simulink library "INP_UNSP_ManOver"  (R2024b)
settings: Solver=VariableStepAuto  StartTime=0.0  StopTime=10.0  RelTol=1e-3
undefined symbols (not defined in the file): INP_UNSP_p_SwtAccUnspFrLeMan_na, INP_UNSP_p_SwtAccUnspFrRiMan_na, INP_UNSP_p_SwtAccUnspReLeMan_na, INP_UNSP_p_SwtAccUnspReRiMan_na, INP_UNSP_s_AccUnspFrLeMan_mps2, INP_UNSP_s_AccUnspFrRiMan_mps2, INP_UNSP_s_AccUnspLoLimFrLe_mps2, INP_UNSP_s_AccUnspLoLimFrRi_mps2, INP_UNSP_s_AccUnspLoLimReLe_mps2, INP_UNSP_s_AccUnspLoLimReRi_mps2, INP_UNSP_s_AccUnspReLeMan_mps2, INP_UNSP_s_AccUnspReRiMan_mps2, INP_UNSP_s_AccUnspUpLimFrLe_mps2, INP_UNSP_s_AccUnspUpLimFrRi_mps2, INP_UNSP_s_AccUnspUpLimReLe_mps2, INP_UNSP_s_AccUnspUpLimReRi_mps2
libraries: simulink x4
settings Model: Creator=blatak  LastModifiedBy=jmbsp

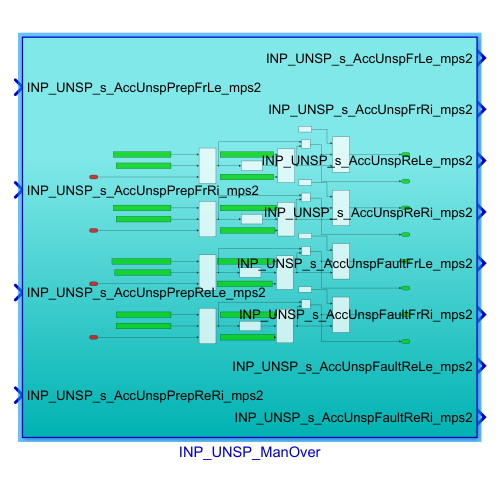
[thumbnail: Simulink's stored preview of the top-level diagram]
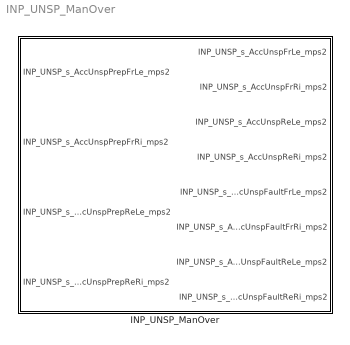
== system INP_UNSP_ManOver ==
  INP_UNSP_ManOver : Subsystem

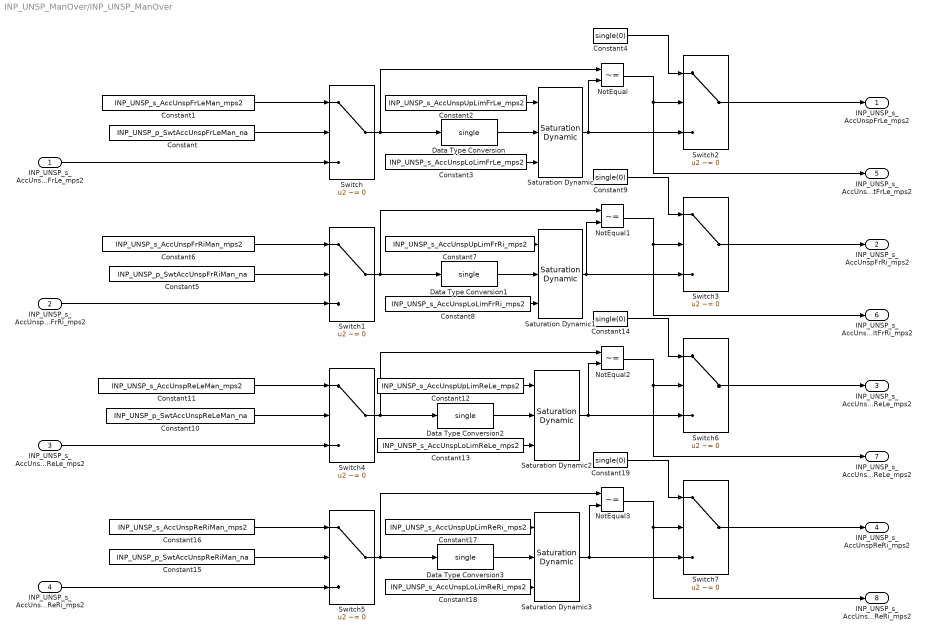
== system INP_UNSP_ManOver/INP_UNSP_ManOver ==
  INP_UNSP_s_AccUnspPrepFrLe_mps2 : Inport
  INP_UNSP_s_AccUnspPrepFrRi_mps2 : Inport  Port=2
  INP_UNSP_s_AccUnspPrepReLe_mps2 : Inport  Port=3
  INP_UNSP_s_AccUnspPrepReRi_mps2 : Inport  Port=4
  Constant : Constant  Description=|  Value=INP_UNSP_p_SwtAccUnspFrLeMan_na
      | Switch for manual override of the longitudinal acceleration value, if 1 instead the measured 
      | value the INP_IMU_p_ALgtVehMan_mps2 is used
  Constant1 : Constant  Description=|  Value=INP_UNSP_s_AccUnspFrLeMan_mps2
      | Value for longitudinal acceleration, which is used if the INP_IMU_p_SwtAXxxVehMan_na
      | is set to 1 instead of the measured value
  Constant10 : Constant  Description=|  Value=INP_UNSP_p_SwtAccUnspReLeMan_na
      | Switch for manual override of the longitudinal acceleration value, if 1 instead the measured 
      | value the INP_IMU_p_ALgtVehMan_mps2 is used
  Constant11 : Constant  Description=|  Value=INP_UNSP_s_AccUnspReLeMan_mps2
      | Value for longitudinal acceleration, which is used if the INP_IMU_p_SwtAXxxVehMan_na
      | is set to 1 instead of the measured value
  Constant12 : Constant  Description=Upper saturation limit for longitudinal acceleration  Value=INP_UNSP_s_AccUnspUpLimReLe_mps2
  Constant13 : Constant  Description=Lower saturation limit for longitudinal acceleration  Value=INP_UNSP_s_AccUnspLoLimReLe_mps2
  Constant{4,9,14,19} (4 alike) : Constant  Value=single(0)
  Constant15 : Constant  Description=|  Value=INP_UNSP_p_SwtAccUnspReRiMan_na
      | Switch for manual override of the longitudinal acceleration value, if 1 instead the measured 
      | value the INP_IMU_p_ALgtVehMan_mps2 is used
  Constant16 : Constant  Description=|  Value=INP_UNSP_s_AccUnspReRiMan_mps2
      | Value for longitudinal acceleration, which is used if the INP_IMU_p_SwtAXxxVehMan_na
      | is set to 1 instead of the measured value
  Constant17 : Constant  Description=Upper saturation limit for longitudinal acceleration  Value=INP_UNSP_s_AccUnspUpLimReRi_mps2
  Constant18 : Constant  Description=Lower saturation limit for longitudinal acceleration  Value=INP_UNSP_s_AccUnspLoLimReRi_mps2
  Constant2 : Constant  Description=Upper saturation limit for longitudinal acceleration  Value=INP_UNSP_s_AccUnspUpLimFrLe_mps2
  Constant3 : Constant  Description=Lower saturation limit for longitudinal acceleration  Value=INP_UNSP_s_AccUnspLoLimFrLe_mps2
  Constant5 : Constant  Description=|  Value=INP_UNSP_p_SwtAccUnspFrRiMan_na
      | Switch for manual override of the longitudinal acceleration value, if 1 instead the measured 
      | value the INP_IMU_p_ALgtVehMan_mps2 is used
  Constant6 : Constant  Description=|  Value=INP_UNSP_s_AccUnspFrRiMan_mps2
      | Value for longitudinal acceleration, which is used if the INP_IMU_p_SwtAXxxVehMan_na
      | is set to 1 instead of the measured value
  Constant7 : Constant  Description=Upper saturation limit for longitudinal acceleration  Value=INP_UNSP_s_AccUnspUpLimFrRi_mps2
  Constant8 : Constant  Description=Lower saturation limit for longitudinal acceleration  Value=INP_UNSP_s_AccUnspLoLimFrRi_mps2
  Data Type Conversion{,1..3} (4 alike) : DataTypeConversion  OutDataTypeStr=single  SaturateOnIntegerOverflow=off  RndMeth=Floor
  NotEqual{,1..3} (4 alike) : RelationalOperator  Operator=~=  OutDataTypeStr=boolean  RndMeth=Simplest  InputSameDT=off
  Saturation Dynamic{,1..3} (4 alike) : simulink/Discontinuities/Saturation Dynamic  OutMin=[]  OutMax=[]  OutDataTypeStr=Inherit: Same as second input  OutDataType=fixdt(1, 16)  OutScaling=2^-10  DoSatur=off
  Switch{,1..7} (8 alike) : Switch  Criteria=u2 ~= 0  SaturateOnIntegerOverflow=off  InputSameDT=off
  INP_UNSP_s_AccUnspFrLe_mps2 : Outport
  INP_UNSP_s_AccUnspFrRi_mps2 : Outport  Port=2
  INP_UNSP_s_AccUnspReLe_mps2 : Outport  Port=3
  INP_UNSP_s_AccUnspReRi_mps2 : Outport  Port=4
  INP_UNSP_s_AccUnspFaultFrLe_mps2 : Outport  Port=5
  INP_UNSP_s_AccUnspFaultFrRi_mps2 : Outport  Port=6
  INP_UNSP_s_AccUnspFaultReLe_mps2 : Outport  Port=7
  INP_UNSP_s_AccUnspFaultReRi_mps2 : Outport  Port=8
  wires:
  INP_UNSP_s_AccUnspPrepReRi_mps2/1 -> Switch5/3
  Data Type Conversion3/1 -> Saturation Dynamic3/2
  NotEqual/1 -> INP_UNSP_s_AccUnspFaultFrLe_mps2/1, Switch2/2
  NotEqual2/1 -> INP_UNSP_s_AccUnspFaultReLe_mps2/1, Switch6/2
  Constant9/1 -> Switch3/1
  Constant6/1 -> Switch1/1
  Constant18/1 -> Saturation Dynamic3/3
  Constant16/1 -> Switch5/1
  Constant10/1 -> Switch4/2
  Switch4/1 -> NotEqual2/1, Data Type Conversion2/1
  Saturation Dynamic1/1 -> Switch3/3, NotEqual1/2
  Constant5/1 -> Switch1/2
  Data Type Conversion2/1 -> Saturation Dynamic2/2
  Saturation Dynamic3/1 -> Switch7/3, NotEqual3/2
  Constant4/1 -> Switch2/1
  Constant2/1 -> Saturation Dynamic/1
  Saturation Dynamic2/1 -> Switch6/3, NotEqual2/2
  Saturation Dynamic/1 -> Switch2/3, NotEqual/2
  INP_UNSP_s_AccUnspPrepFrRi_mps2/1 -> Switch1/3
  Constant/1 -> Switch/2
  Switch5/1 -> NotEqual3/1, Data Type Conversion3/1
  Switch1/1 -> NotEqual1/1, Data Type Conversion1/1
  Switch7/1 -> INP_UNSP_s_AccUnspReRi_mps2/1
  Data Type Conversion1/1 -> Saturation Dynamic1/2
  Constant17/1 -> Saturation Dynamic3/1
  Constant14/1 -> Switch6/1
  Constant12/1 -> Saturation Dynamic2/1
  NotEqual1/1 -> INP_UNSP_s_AccUnspFaultFrRi_mps2/1, Switch3/2
  Constant3/1 -> Saturation Dynamic/3
  Constant19/1 -> Switch7/1
  Constant1/1 -> Switch/1
  INP_UNSP_s_AccUnspPrepFrLe_mps2/1 -> Switch/3
  Switch3/1 -> INP_UNSP_s_AccUnspFrRi_mps2/1
  Constant15/1 -> Switch5/2
  Constant7/1 -> Saturation Dynamic1/1
  NotEqual3/1 -> INP_UNSP_s_AccUnspFaultReRi_mps2/1, Switch7/2
  Constant11/1 -> Switch4/1
  Data Type Conversion/1 -> Saturation Dynamic/2
  Constant13/1 -> Saturation Dynamic2/3
  Constant8/1 -> Saturation Dynamic1/3
  Switch6/1 -> INP_UNSP_s_AccUnspReLe_mps2/1
  Switch/1 -> NotEqual/1, Data Type Conversion/1
  INP_UNSP_s_AccUnspPrepReLe_mps2/1 -> Switch4/3
  Switch2/1 -> INP_UNSP_s_AccUnspFrLe_mps2/1
